simulink subsystem "Throttle_Map"  (R2023b)
settings: Solver=VariableStepAuto  StartTime=0.0  StopTime=10.0  RelTol=1e-3
values from neighbouring files (symbols this model uses):
  dk_grid = max(k_grid_max - k_grid_min,0)    [Motor_Tables.m]
  k_grid_min = feval(fitresult,voltage_grid_min,rpm_grid_min)    [Motor_Tables.m]
  rpm_sweep_min = linspace(0, max(motor_constants(1,:)), RPM_resolution)    [Motor_Tables.m]
  voltage_sweep_min = linspace(min(voltages), max(voltages), V_resolution)    [Motor_Tables.m]
undefined symbols (not defined in the file or in its folder): sim
settings Model: Creator=Inver  LastModifiedBy=Inver

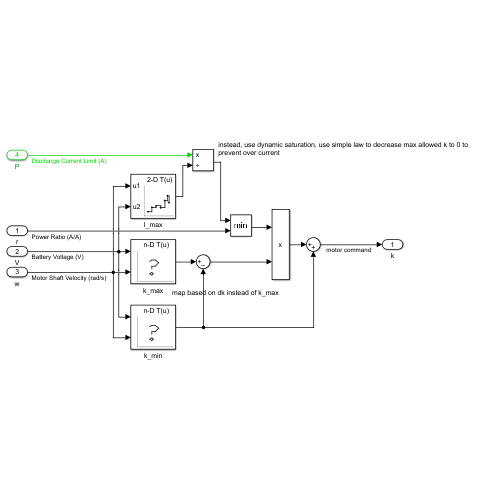
[thumbnail: Simulink's stored preview of the top-level diagram]
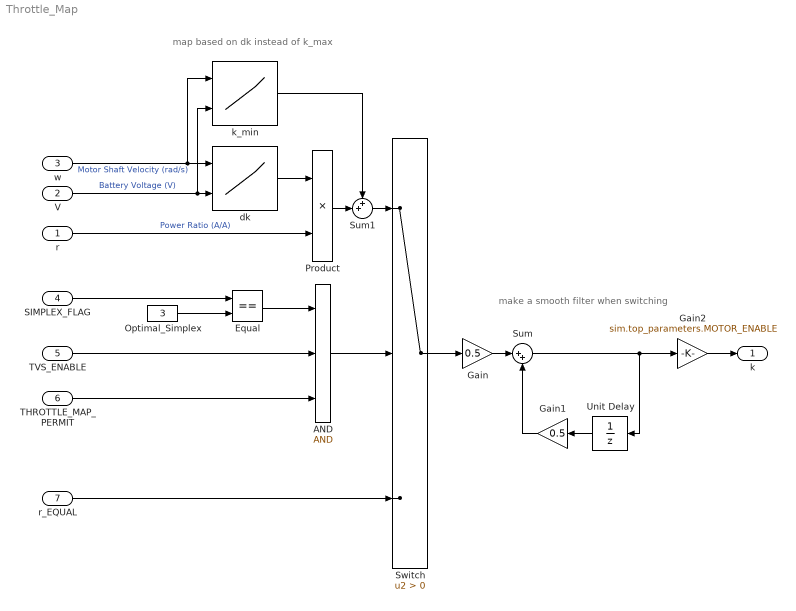
== system Throttle_Map ==
  note: map based on dk instead of k_max
  note: make a smooth filter when switching
  r : Inport
  V : Inport  Port=2
  w : Inport  Port=3
  SIMPLEX_FLAG : Inport  Port=4
  TVS_ENABLE : Inport  Port=5
  THROTTLE_MAP_PERMIT : Inport  Port=6
  r_EQUAL : Inport  Port=7
  AND : Logic  Inputs=3  IconShape=distinctive  AllPortsSameDT=off  OutDataTypeStr=boolean
  Equal : RelationalOperator  Operator===  OutDataTypeStr=boolean  RndMeth=Simplest  InputSameDT=off
  Gain : Gain  Gain=0.5
  Gain1 : Gain  Gain=0.5
  Gain2 : Gain  Gain=sim.top_parameters.MOTOR_ENABLE
  Optimal_Simplex : Constant  Value=3
  Product : Product
  Sum : Sum  Inputs=|++
  Sum1 : Sum  Inputs=++|
  Switch : Switch  Criteria=u2 > Threshold  SaturateOnIntegerOverflow=off  InputSameDT=off
  Unit Delay : UnitDelay  SampleTime=-1  HasFrameUpgradeWarning=on
  dk : Lookup_n-D  LookupTableObject=''  BreakpointsForDimension1=rpm_sweep_min  BreakpointsForDimension2=voltage_sweep_min  BreakpointsForDimension1FirstPoint=10  BreakpointsForDimension2FirstPoint=10  BreakpointsForDimension1Spacing=12  BreakpointsForDimension2Spacing=12  IndexSearchMethod=Evenly spaced points  Table=dk_grid  ExtrapMethod=Clip  DiagnosticForOutOfRangeInput=Error  InternalRulePriority=Speed  RndMeth=Simplest
      settings: InputPortMap=u0,u1
  k_min : Lookup_n-D  LookupTableObject=''  BreakpointsForDimension1=rpm_sweep_min  BreakpointsForDimension2=voltage_sweep_min  BreakpointsForDimension1FirstPoint=10  BreakpointsForDimension2FirstPoint=10  BreakpointsForDimension1Spacing=12  BreakpointsForDimension2Spacing=12  IndexSearchMethod=Evenly spaced points  Table=k_grid_min  ExtrapMethod=Clip  DiagnosticForOutOfRangeInput=Error  InternalRulePriority=Speed  RndMeth=Simplest
      settings: InputPortMap=u0,u1
  k : Outport
  wires:
  w/1 -> dk/1, k_min/1  "Motor Shaft Velocity (rad/s)"
  V/1 -> dk/2, k_min/2  "Battery Voltage (V)"
  r/1 -> Product/2  "Power Ratio (A/A)"
  Sum1/1 -> Switch/1
  k_min/1 -> Sum1/1
  dk/1 -> Product/1
  Switch/1 -> Gain/1
  Gain1/1 -> Sum/2
  Gain/1 -> Sum/1
  Sum/1 -> Unit Delay/1, Gain2/1
  Unit Delay/1 -> Gain1/1
  Product/1 -> Sum1/2
  Gain2/1 -> k/1
  THROTTLE_MAP_PERMIT/1 -> AND/3
  TVS_ENABLE/1 -> AND/2
  SIMPLEX_FLAG/1 -> Equal/1
  AND/1 -> Switch/2
  Optimal_Simplex/1 -> Equal/2
  Equal/1 -> AND/1
  r_EQUAL/1 -> Switch/3
